simulink model "sl_drivepoint_Scripts"  (R2016b)
settings: Solver=ode45  StartTime=0.0  StopTime=60  RelTol=1e-3  EnableMultiTasking=on
libraries: simulink x1, roblocks x1
settings Model: Creator=pic  LastModifiedBy=Antonio
settings DataIOCC: SaveFormat=Array  ReturnWorkspaceOutputs=on  TimeSaveName=t  OutputSaveName=y
settings OptimizationCC: ExpressionDepthLimit=2147483647  LifeSpan=inf
settings DebuggingCC: UnderspecifiedInitializationDetection=Classic  MergeDetectMultiDrivingBlocksExec=none  AllowSymbolicDim=off  StateNameClashWarn=warning  SFUnexpectedBacktrackingDiag=warning  SFNoUnconditionalDefaultTransitionDiag=warning  SFExecutionAtInitializationDiag=none
settings HardwareCC: ProdBitPerPointer=32  ProdBitPerSizeT=32  ProdBitPerPtrDiffT=32  ProdLargestAtomicFloat=None  ProdIntDivRoundTo=Undefined  ProdEndianess=Unspecified  ProdWordSize=32  ProdHWDeviceType=32-bit Generic
settings ModelReferenceCC: PropagateSignalLabelsOutOfModel=off
settings GRTTargetCC: TargetLangStandard=C89/C90 (ANSI)  GeneratePreprocessorConditionals=Disable all  CombineOutputUpdateFcns=off  GRTInterface=on
settings ConfigComp: CovMetricSettings=dw  CovHtmlReporting=on  CovSaveCumulativeToWorkspaceVar=on  CovSaveSingleToWorkspaceVar=on  CovExternalEMLEnable=off

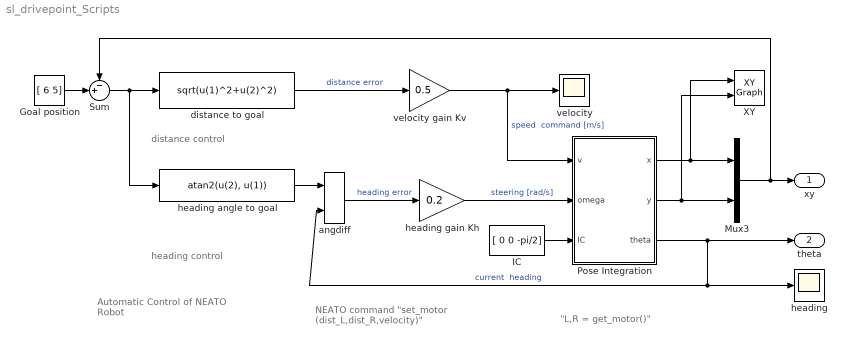
== system sl_drivepoint_Scripts ==
  note: Automatic Control of
      | NEATO Robot
  note: NEATO command
      | "set_motor (dist_L,dist_R,velocity)"
  note: distance control
  note: heading control
  note: "L,R = get_motor()"
  Goal position : Constant  Value=[ 6 5]
  IC : Constant  Value=[ 0 0 -pi/2]
  Mux3 : Mux  Inputs=2
  Pose Integration : Subsystem  AncestorBlock=roblocks/Vehicles/Unicycle  mask{accel=0.3, vlim=1, alim=0.5, L=0.52, x0=[0, 0, -pi/2], a=0.26}
      mask prompts: accel "Acceleration"; vlim "Velocity limit"; alim "Steering limits"; L "Wheel base"; x0 "Initial state (x, y, theta)"; a "Coordinate frame shift (a)"
      mask help: Kino-dynamic model of bicycle vehicle
      mask Help:
      | Kino-dynamic model of bicycle vehicle, also known as Ackermann vehicle
      | model.
      | 
      | <b>Parameters::</b>
      | 
      | Acceleration (1x1)   Vehicle acceleration limit [m/s2]
      | Velocity limit (1x1)  Vehicle speed limit [m/s]
      | Steering limits (1x1) Steering angle limit [rad]
      | Initial state (1x3) Initial state (x, y, theta)
      | Handbrake (1x1) Vehicle cannot move if non-zero
      | 
      | <b>Inputs::</b>
      | 
      | v (1x1) velocity demand [m/s]
      | gamma (1x1) steering angle [rad]
      | 
      | <b>Outputs::</b>
      | 
      | x (1x1) x-coordinate in world frame [m]
      | y (1x1) x-coordinate in world frame [m]
      | theta (1x1) heading angle in world frame [rad]
      | 
      | 
      | <b>Notes::</b>
      | 
      | - Steering limit is symmetric between -limit and +limit
      | - Same dynamic model as the Toolbox class Vehicle.
      mask Display:
      | port_label('input', 1, 'v')
      | port_label('input', 2, '\omega', 'texmode', 'on')
      | port_label('input', 3, 'x0')
      | port_label('output', 1, 'x')
      | port_label('output', 2, 'y')
      | port_label('output', 3, '\theta', 'texmode', 'on')
  Sum : Sum  Inputs=-+|
  XY : simulink/Sinks/XY Graph  xmin=-5  xmax=10  ymin=-5  ymax=10  st=-1
  angdiff : roblocks/Toolbox/angdiff
  distance to goal : Fcn  Expr=sqrt(u(1)^2+u(2)^2)
  heading : Scope
  heading angle to goal : Fcn  Expr=atan2(u(2), u(1))
  heading gain Kh : Gain  Gain=0.2
  velocity : Scope
  velocity gain Kv : Gain  Gain=0.5
  xy : Outport
  "theta " : Outport  Port=2
  wires:
  Pose Integration/1(x) -> XY/1, Mux3/1
  Pose Integration/2(y) -> Mux3/2, XY/2
  Mux3/1 -> Sum/1, xy/1
  Sum/1 -> heading angle to goal/1, distance to goal/1
  distance to goal/1 -> velocity gain Kv/1  "distance error"
  heading angle to goal/1 -> angdiff/1
  Pose Integration/3(theta) -> "theta "/1, angdiff/2, heading/1  "current  heading"
  angdiff/1 -> heading gain Kh/1  "heading error"
  velocity gain Kv/1 -> Pose Integration/1(v), velocity/1  "speed  command [m/s]"
  Goal position/1 -> Sum/2
  heading gain Kh/1 -> Pose Integration/2(omega)  "steering [rad/s]"
  IC/1 -> Pose Integration/3(IC)

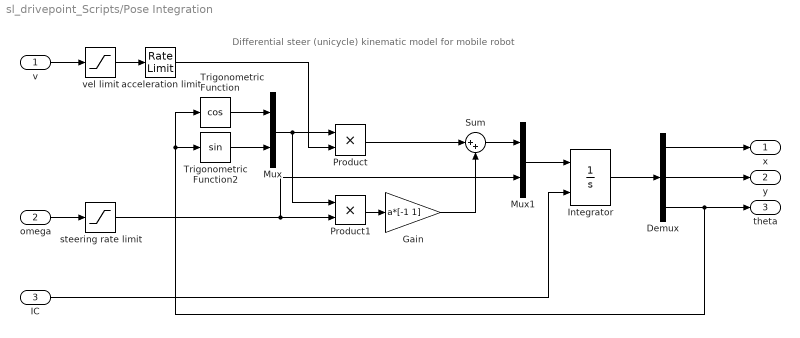
== system sl_drivepoint_Scripts/Pose Integration ==
  note: Differential steer (unicycle) kinematic model for mobile robot
  v : Inport
  omega : Inport  Port=2
  IC : Inport  Port=3
  Demux : Demux  Outputs=3
  Gain : Gain  Gain=a*[-1 1]
  Integrator : Integrator  InitialConditionSource=external  InitialCondition=[0 0 -pi]
  Mux : Mux  Inputs=2
  Mux1 : Mux  Inputs=2
  Product : Product  RndMeth=Zero
  Product1 : Product  RndMeth=Zero
  Sum : Sum  Inputs=|++
  Trigonometric Function : Trigonometry  Operator=cos
  Trigonometric Function2 : Trigonometry
  acceleration limit : RateLimiter  RisingSlewLimit=accel  FallingSlewLimit=-accel  SampleTimeMode=inherited
  steering rate limit : Saturate  UpperLimit=alim  LowerLimit=-alim
  vel limit : Saturate  UpperLimit=vlim  LowerLimit=-vlim
  x : Outport
  y : Outport  Port=2
  theta : Outport  Port=3
  wires:
  Gain/1 -> Sum/2
  Product1/1 -> Gain/1
  Sum/1 -> Mux1/1
  Product/1 -> Sum/1
  Mux1/1 -> Integrator/1
  steering rate limit/1 -> Product1/2, Mux1/2
  Trigonometric Function2/1 -> Mux/2
  vel limit/1 -> acceleration limit/1
  Mux/1 -> Product/1, Product1/1
  v/1 -> vel limit/1
  omega/1 -> steering rate limit/1
  Demux/2 -> y/1
  Demux/1 -> x/1
  Demux/3 -> Trigonometric Function2/1, Trigonometric Function/1, theta/1
  Integrator/1 -> Demux/1
  acceleration limit/1 -> Product/2
  Trigonometric Function/1 -> Mux/1
  IC/1 -> Integrator/2
